simulink model "X31dynamics_03_controller_NDI_MG"  (R2014b)
settings: Solver=ode45  StartTime=0.0  StopTime=30  FixedStep=0.01  RelTol=1e-3
InitFcn:
  | X31dynamics_03_controller_NDI_init
values from neighbouring files (symbols this model uses):
  X31_controller = evalin('base','X31_controller')    [X31dynamics_03_controller_MG_iter_3_2_9_10.m]
undefined symbols (not defined in the file or in its folder): sigbuilder_block, X31_initC, X31_MnvrGen
libraries: simulink x17, QuaternionLib x3
(part 2 of 2)

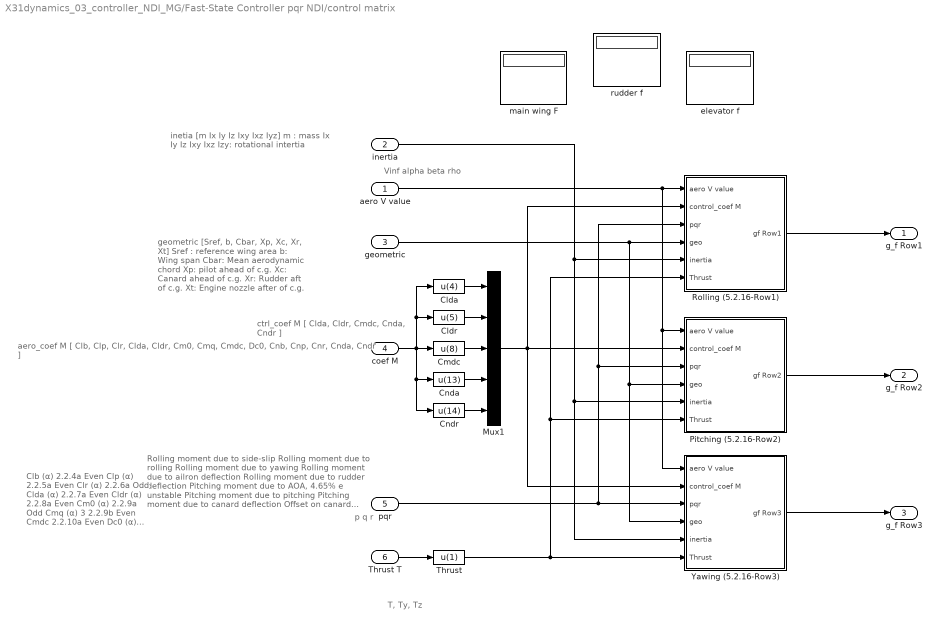
== system X31dynamics_03_controller_NDI_MG/Fast-State Controller pqr NDI/control matrix ==
  note: Vinf alpha beta rho
  note: p q r
  note: geometric
      |  [Sref, b, Cbar, Xp, Xc, Xr, Xt]
      |
      | Sref : reference wing area
      | b: Wing span
      | Cbar: Mean aerodynamic chord
      | Xp: pilot ahead of c.g.
      | Xc: Canard ahead of c.g.
      | Xr: Rudder aft of c.g.
      | Xt: Engine nozzle after of c.g.
  note: Rolling moment due to side-slip
      | Rolling moment due to rolling
      | Rolling moment due to yawing
      | Rolling moment due to ailron deflection
      | Rolling moment due to rudder deflection
      |
      | Pitching moment due to AOA, 4.65% e unstable
      | Pitching moment due to pitching
      | Pitching moment due to canard deflection
      | Offset on canard deflection
      |
      | Yawing moment due to side-slip
      | Yawing moment due to rolling
      | Yawing moment due to yawing
      | Yawing moment due to ailron deflection
      | Yawing moment due to rudder deflection
  note: Clb    (α) 2.2.4a Even
      | Clp    (α) 2.2.5a Even
      | Clr     (α) 2.2.6a Odd
      | Clda  (α) 2.2.7a Even
      | Cldr   (α) 2.2.8a Even
      |
      | Cm0  (α) 2.2.9a Odd
      | Cmq  (α) 3 2.2.9b Even
      | Cmdc      2.2.10a Even
      | Dc0   (α) 2.2.2/10b Odd
      |
      | Cnb  (α) 2.2.4b Even
      | Cnp  (α) 2.2.5b Odd
      | Cnr   (α) 2.2.6b Even
      | Cnda(α) 2.2.7b Even
      | Cndr (α) 2.2.8b Even
  note: aero_coef M
      | [ Clb, Clp, Clr, Clda, Cldr, Cm0, Cmq, Cmdc, Dc0, Cnb, Cnp, Cnr, Cnda, Cndr ]
  note: inetia
      | [m Ix Iy Iz Ixy Ixz Iyz]
      | m : mass
      | Ix Iy Iz Ixy Ixz Izy: rotational intertia
  note: ctrl_coef M
      | [ Clda, Cldr, Cmdc, Cnda, Cndr ]
  note: T, Ty, Tz
  aero V value : Inport
  inertia : Inport  Port=2
  geometric : Inport  Port=3
  coef M : Inport  Port=4
  pqr : Inport  Port=5
  Thrust T : Inport  Port=6
  Clda : Fcn  Expr=u(4)
  Cldr : Fcn  Expr=u(5)
  Cmdc : Fcn  Expr=u(8)
  Cnda : Fcn  Expr=u(13)
  Cndr : Fcn  Expr=u(14)
  Mux1 : Mux  Inputs=5
  Pitching (5.2.16-Row2) : Subsystem
  Rolling (5.2.16-Row1) : Subsystem
  Thrust : Fcn  Expr=u(1)
  Yawing (5.2.16-Row3) : Subsystem
  elevator f : Display
  main wing F : Display
  rudder f : Display
  g_f Row1 : Outport
  g_f Row2 : Outport  Port=2
  g_f Row3 : Outport  Port=3
  wires:
  pqr/1 -> Yawing (5.2.16-Row3)/3(pqr), Pitching (5.2.16-Row2)/3(pqr), Rolling (5.2.16-Row1)/3(pqr)
  aero V value/1 -> Yawing (5.2.16-Row3)/1(aero V value), Pitching (5.2.16-Row2)/1(aero V value), Rolling (5.2.16-Row1)/1(aero V value)
  coef M/1 -> Clda/1, Cldr/1, Cndr/1, Cnda/1, Cmdc/1
  Mux1/1 -> Yawing (5.2.16-Row3)/2(control_coef M), Pitching (5.2.16-Row2)/2(control_coef M), Rolling (5.2.16-Row1)/2(control_coef M)
  geometric/1 -> Yawing (5.2.16-Row3)/4(geo), Pitching (5.2.16-Row2)/4(geo), Rolling (5.2.16-Row1)/4(geo)
  Clda/1 -> Mux1/1
  Cldr/1 -> Mux1/2
  Cmdc/1 -> Mux1/3
  Cnda/1 -> Mux1/4
  Cndr/1 -> Mux1/5
  Thrust T/1 -> Thrust/1
  inertia/1 -> Pitching (5.2.16-Row2)/5(inertia), Yawing (5.2.16-Row3)/5(inertia), Rolling (5.2.16-Row1)/5(inertia)
  Yawing (5.2.16-Row3)/1(gf Row3) -> g_f Row3/1
  Pitching (5.2.16-Row2)/1(gf Row2) -> g_f Row2/1
  Rolling (5.2.16-Row1)/1(gf Row1) -> g_f Row1/1
  Thrust/1 -> Yawing (5.2.16-Row3)/6(Thrust), Pitching (5.2.16-Row2)/6(Thrust), Rolling (5.2.16-Row1)/6(Thrust)

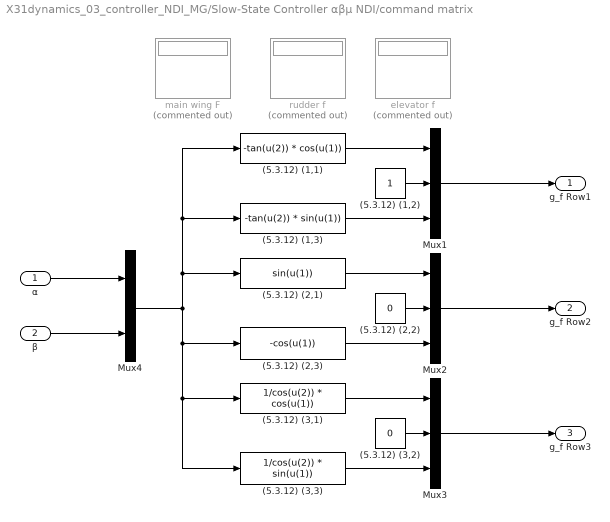
== system X31dynamics_03_controller_NDI_MG/Slow-State Controller αβμ NDI/command matrix ==
  α : Inport
  β : Inport  Port=2
  (5.3.12) (1,1) : Fcn  Expr=-tan(u(2)) * cos(u(1))
  (5.3.12) (1,2) : Constant
  (5.3.12) (1,3) : Fcn  Expr=-tan(u(2)) * sin(u(1))
  (5.3.12) (2,1) : Fcn  Expr=sin(u(1))
  (5.3.12) (2,2) : Constant  Value=0
  (5.3.12) (2,3) : Fcn  Expr=-cos(u(1))
  (5.3.12) (3,1) : Fcn  Expr=1/cos(u(2)) * cos(u(1))
  (5.3.12) (3,2) : Constant  Value=0
  (5.3.12) (3,3) : Fcn  Expr=1/cos(u(2)) * sin(u(1))
  Mux1 : Mux  Inputs=3
  Mux2 : Mux  Inputs=3
  Mux3 : Mux  Inputs=3
  Mux4 : Mux  Inputs=2
  elevator f : Display  Commented=on
  main wing F : Display  Commented=on
  rudder f : Display  Commented=on
  g_f Row1 : Outport
  g_f Row2 : Outport  Port=2
  g_f Row3 : Outport  Port=3
  wires:
  Mux3/1 -> g_f Row3/1
  Mux2/1 -> g_f Row2/1
  Mux1/1 -> g_f Row1/1
  α/1 -> Mux4/1
  β/1 -> Mux4/2
  (5.3.12) (3,2)/1 -> Mux3/2
  (5.3.12) (2,2)/1 -> Mux2/2
  (5.3.12) (1,2)/1 -> Mux1/2
  Mux4/1 -> (5.3.12) (1,3)/1, (5.3.12) (1,1)/1, (5.3.12) (2,1)/1, (5.3.12) (3,3)/1, (5.3.12) (3,1)/1, (5.3.12) (2,3)/1
  (5.3.12) (1,1)/1 -> Mux1/1
  (5.3.12) (1,3)/1 -> Mux1/3
  (5.3.12) (2,1)/1 -> Mux2/1
  (5.3.12) (2,3)/1 -> Mux2/3
  (5.3.12) (3,1)/1 -> Mux3/1
  (5.3.12) (3,3)/1 -> Mux3/3

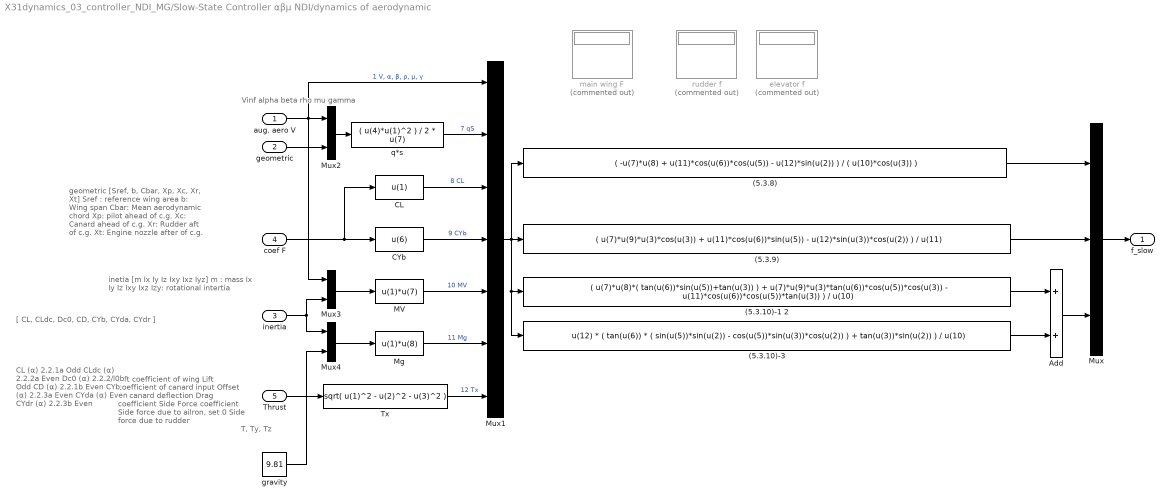
== system X31dynamics_03_controller_NDI_MG/Slow-State Controller αβμ NDI/dynamics of aerodynamic ==
  note: Vinf alpha beta rho mu gamma
  note: geometric
      |  [Sref, b, Cbar, Xp, Xc, Xr, Xt]
      |
      | Sref : reference wing area
      | b: Wing span
      | Cbar: Mean aerodynamic chord
      | Xp: pilot ahead of c.g.
      | Xc: Canard ahead of c.g.
      | Xr: Rudder aft of c.g.
      | Xt: Engine nozzle after of c.g.
  note: Lift coefficient of wing
      | Lift coefficient of canard input
      | Offset on canard deflection
      | Drag coefficient
      | Side Force coefficient
      | Side force due to ailron, set 0
      | Side force due to rudder
  note: CL     (α) 2.2.1a Odd
      | CLdc (α)  2.2.2a Even
      | Dc0   (α)  2.2.2/l0b Odd
      | CD     (α)  2.2.1b Even
      | CYb   (α) 2.2.3a Even
      | CYda (α)            Even
      | CYdr  (α) 2.2.3b Even
  note: [ CL, CLdc, Dc0, CD, CYb, CYda, CYdr ]
  note: T, Ty, Tz
  note: inetia
      | [m Ix Iy Iz Ixy Ixz Iyz]
      | m : mass
      | Ix Iy Iz Ixy Ixz Izy: rotational intertia
  aug. aero V : Inport
  geometric : Inport  Port=2
  inertia : Inport  Port=3
  coef F : Inport  Port=4
  Thrust : Inport  Port=5
  (5.3.10)-1 2 : Fcn  Expr="( u(7)*u(8)*( tan(u(6))*sin(u(5))+tan(u(3)) ) + u(7)*u(9)*u(3)*tan(u(6))*cos(u(5))*cos(u(3)) - u(11)*cos(u(6))*cos(u(5))*tan(u(3)) ) /  u(10)"
  (5.3.10)-3 : Fcn  Expr=u(12) * ( tan(u(6)) * ( sin(u(5))*sin(u(2)) - cos(u(5))*sin(u(3))*cos(u(2)) ) + tan(u(3))*sin(u(2)) ) / u(10)
  (5.3.8) : Fcn  Expr=( -u(7)*u(8) + u(11)*cos(u(6))*cos(u(5)) - u(12)*sin(u(2)) ) / ( u(10)*cos(u(3)) )
  (5.3.9) : Fcn  Expr=( u(7)*u(9)*u(3)*cos(u(3)) + u(11)*cos(u(6))*sin(u(5)) - u(12)*sin(u(3))*cos(u(2)) ) / u(11)
  Add : Sum
  CL : Fcn  Expr=u(1)
  CYb : Fcn  Expr=u(6)
  MV : Fcn  Expr=u(1)*u(7)
  Mg : Fcn  Expr=u(1)*u(8)
  Mux : Mux  Inputs=3
  Mux1 : Mux  Inputs=7
  Mux2 : Mux  Inputs=2
  Mux3 : Mux  Inputs=2
  Mux4 : Mux  Inputs=2
  Tx : Fcn  Expr=sqrt( u(1)^2 - u(2)^2 - u(3)^2 )
  elevator f : Display  Commented=on
  gravity : Constant  Value=9.81
  main wing F : Display  Commented=on
  q*s : Fcn  Expr=( u(4)*u(1)^2 ) / 2 * u(7)
  rudder f : Display  Commented=on
  f_slow : Outport
  wires:
  Mux/1 -> f_slow/1
  aug. aero V/1 -> Mux2/1, Mux1/1, Mux3/1  "1 V, α, β, ρ, μ, γ"
  coef F/1 -> CL/1, CYb/1
  geometric/1 -> Mux2/2
  q*s/1 -> Mux1/2  "7 qS"
  (5.3.10)-1 2/1 -> Add/1
  (5.3.8)/1 -> Mux/1
  (5.3.9)/1 -> Mux/2
  Mux3/1 -> MV/1
  Thrust/1 -> Tx/1
  Tx/1 -> Mux1/7  "12 Tx"
  MV/1 -> Mux1/5  "10 MV"
  CYb/1 -> Mux1/4  "9 CYb"
  CL/1 -> Mux1/3  "8 CL"
  Mux1/1 -> (5.3.8)/1, (5.3.9)/1, (5.3.10)-3/1, (5.3.10)-1 2/1
  Mux2/1 -> q*s/1
  inertia/1 -> Mux4/1, Mux3/2
  Mg/1 -> Mux1/6  "11 Mg"
  Mux4/1 -> Mg/1
  gravity/1 -> Mux4/2
  (5.3.10)-3/1 -> Add/2
  Add/1 -> Mux/3

== system X31dynamics_03_controller_NDI_MG/Fast-State Controller pqr NDI/aerodynamic Moment/Pitching coefficient (5.2.14) ==
  note: 9 p q r
  note: 1 Vinf alpha beta rho
  note: 12 Sref, b, Cbar, Xp, Xc, Xr, Xt
  note: 5 Cm0, Cmq, Cmdc, Dc0
  aero V value : Inport
  aero_coef Mb : Inport  Port=2
  pqr : Inport  Port=3
  geo : Inport  Port=4
  Add : Sum
  Aero : Display
  Mux : Mux
  ail prop F body : Display
  main wing F : Display
  pitching (5.2.14-2) : Fcn  Expr=u(6)* u(10)*u(14) / (2*u(1))
  stateR 2 : Display
  static stability (5.2.14-1) : Fcn  Expr=u(5)
  Cm : Outport
  wires:
  aero_coef Mb/1 -> Mux/2
  Mux/1 -> static stability (5.2.14-1)/1, pitching (5.2.14-2)/1
  aero V value/1 -> Mux/1
  pqr/1 -> Mux/3
  pitching (5.2.14-2)/1 -> Add/2
  static stability (5.2.14-1)/1 -> Add/1
  Add/1 -> Cm/1
  geo/1 -> Mux/4

== system X31dynamics_03_controller_NDI_MG/Fast-State Controller pqr NDI/aerodynamic Moment/Rolling coefficient (5.2.13) ==
  note: 10 p q r
  note: 1 Vinf alpha beta rho
  note: 5 Clb, Clp, Clr, Clda, Cldr
  note: 13 Sref, b, Cbar, Xp, Xc, Xr, Xt
  aero V value : Inport
  aero_coef M : Inport  Port=2
  pqr : Inport  Port=3
  geo : Inport  Port=4
  Add : Sum  Inputs=+++
  Aero : Display  Commented=on
  Mux : Mux
  ail prop F body : Display  Commented=on
  main wing F : Display  Commented=on
  rolling (5.2.13-2) : Fcn  Expr=u(6)* u(10)*u(14) / (2*u(1))
  sideslip (5.2.13-1) : Fcn  Expr=u(5)*u(3)
  stateR 2 : Display  Commented=on
  yawing (5.2.13-3) : Fcn  Expr=u(7)* u(12)*u(14) / (2*u(1))
  Cl hat : Outport
  wires:
  aero_coef M/1 -> Mux/2
  Mux/1 -> sideslip (5.2.13-1)/1, rolling (5.2.13-2)/1, yawing (5.2.13-3)/1
  aero V value/1 -> Mux/1
  pqr/1 -> Mux/3
  geo/1 -> Mux/4
  yawing (5.2.13-3)/1 -> Add/3
  rolling (5.2.13-2)/1 -> Add/2
  sideslip (5.2.13-1)/1 -> Add/1
  Add/1 -> Cl hat/1

== system X31dynamics_03_controller_NDI_MG/Fast-State Controller pqr NDI/aerodynamic Moment/Yawing coefficient (5.2.15) ==
  note: 10 p q r
  note: 1 Vinf alpha beta rho
  note: 13 Sref, b, Cbar, Xp, Xc, Xr, Xt
  note: 5 Cnb, Cnp, Cnr, Cnda, Cndr
  aero V value : Inport
  aero_coef M : Inport  Port=2
  pqr : Inport  Port=3
  geo : Inport  Port=4
  Add : Sum  Inputs=+++
  Aero : Display
  Mux : Mux
  ail prop F body : Display
  main wing F : Display
  rolling (5.2.15-2) : Fcn  Expr=u(6)* u(10)*u(14) / (2*u(1))
  sideslip (5.2.15-1) : Fcn  Expr=u(5)*u(3)
  stateR 2 : Display
  yawing (5.2.15-3) : Fcn  Expr=u(7)* u(10)*u(12) / (2*u(1))
  Cn : Outport
  wires:
  aero_coef M/1 -> Mux/2
  Mux/1 -> ail prop F body/1, sideslip (5.2.15-1)/1, rolling (5.2.15-2)/1, yawing (5.2.15-3)/1
  aero V value/1 -> stateR 2/1, Mux/1
  pqr/1 -> Mux/3
  geo/1 -> Mux/4
  yawing (5.2.15-3)/1 -> Add/3
  rolling (5.2.15-2)/1 -> main wing F/1, Add/2
  sideslip (5.2.15-1)/1 -> Add/1
  Add/1 -> Cn/1

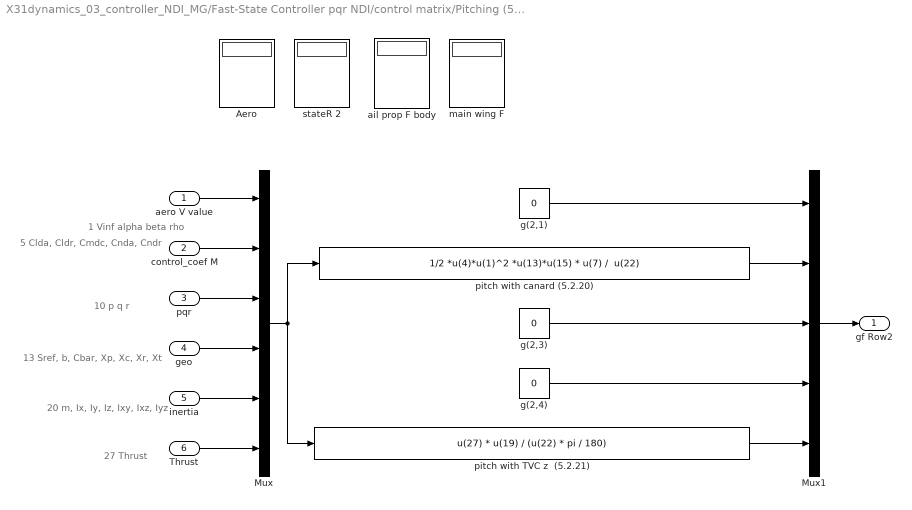
== system X31dynamics_03_controller_NDI_MG/Fast-State Controller pqr NDI/control matrix/Pitching (5.2.16-Row2) ==
  note: 27 Thrust
  note: 10 p q r
  note: 1 Vinf alpha beta rho
  note: 13 Sref, b, Cbar, Xp, Xc, Xr, Xt
  note: 20 m, Ix, Iy, Iz, Ixy, Ixz, Iyz
  note: 5 Clda, Cldr, Cmdc, Cnda, Cndr
  aero V value : Inport
  control_coef M : Inport  Port=2
  pqr : Inport  Port=3
  geo : Inport  Port=4
  inertia : Inport  Port=5
  Thrust : Inport  Port=6
  Aero : Display
  Mux : Mux  Inputs=6
  Mux1 : Mux  Inputs=5
  ail prop F body : Display
  g(2,1) : Constant  Value=0
  g(2,3) : Constant  Value=0
  g(2,4) : Constant  Value=0
  main wing F : Display
  pitch with TVC z  (5.2.21) : Fcn  Expr=u(27) * u(19) / (u(22) * pi / 180)
  pitch with canard (5.2.20) : Fcn  Expr="1/2 *u(4)*u(1)^2 *u(13)*u(15) * u(7) /  u(22)"
  stateR 2 : Display
  gf Row2 : Outport
  wires:
  control_coef M/1 -> Mux/2
  Mux/1 -> pitch with TVC z  (5.2.21)/1, pitch with canard (5.2.20)/1
  aero V value/1 -> Mux/1
  pqr/1 -> Mux/3
  geo/1 -> Mux/4
  pitch with TVC z  (5.2.21)/1 -> Mux1/5
  g(2,3)/1 -> Mux1/3
  pitch with canard (5.2.20)/1 -> Mux1/2
  Mux1/1 -> gf Row2/1
  g(2,1)/1 -> Mux1/1
  g(2,4)/1 -> Mux1/4
  inertia/1 -> Mux/5
  Thrust/1 -> Mux/6

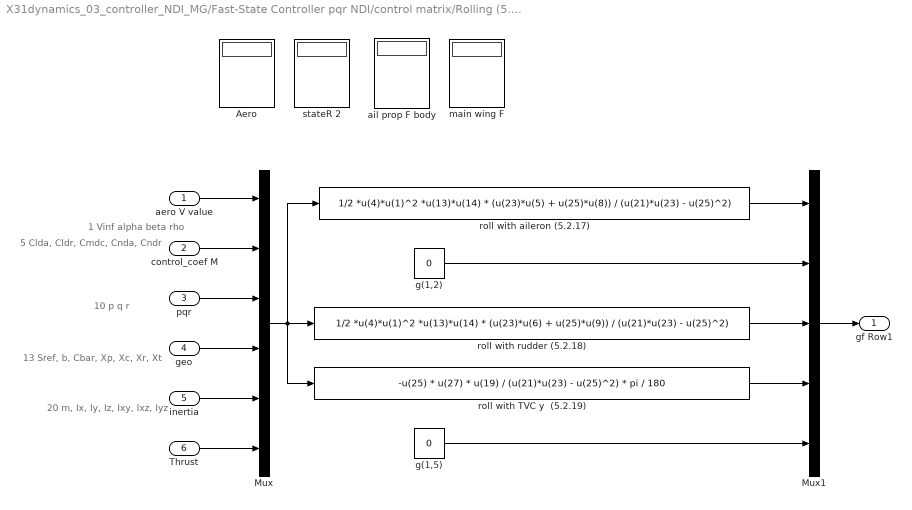
== system X31dynamics_03_controller_NDI_MG/Fast-State Controller pqr NDI/control matrix/Rolling (5.2.16-Row1) ==
  note: 10 p q r
  note: 1 Vinf alpha beta rho
  note: 13 Sref, b, Cbar, Xp, Xc, Xr, Xt
  note: 20 m, Ix, Iy, Iz, Ixy, Ixz, Iyz
  note: 5 Clda, Cldr, Cmdc, Cnda, Cndr
  aero V value : Inport
  control_coef M : Inport  Port=2
  pqr : Inport  Port=3
  geo : Inport  Port=4
  inertia : Inport  Port=5
  Thrust : Inport  Port=6
  Aero : Display
  Mux : Mux  Inputs=6
  Mux1 : Mux  Inputs=5
  ail prop F body : Display
  g(1,2) : Constant  Value=0
  g(1,5) : Constant  Value=0
  main wing F : Display
  roll with TVC y  (5.2.19) : Fcn  Expr=-u(25) * u(27) * u(19) / (u(21)*u(23) - u(25)^2) * pi / 180
  roll with aileron (5.2.17) : Fcn  Expr=1/2 *u(4)*u(1)^2 *u(13)*u(14) * (u(23)*u(5) + u(25)*u(8)) / (u(21)*u(23) - u(25)^2)
  roll with rudder (5.2.18) : Fcn  Expr=1/2 *u(4)*u(1)^2 *u(13)*u(14) * (u(23)*u(6) + u(25)*u(9)) / (u(21)*u(23) - u(25)^2)
  stateR 2 : Display
  gf Row1 : Outport
  wires:
  control_coef M/1 -> Mux/2
  Mux/1 -> roll with rudder (5.2.18)/1, roll with TVC y  (5.2.19)/1, roll with aileron (5.2.17)/1
  aero V value/1 -> Mux/1
  pqr/1 -> Mux/3
  geo/1 -> Mux/4
  roll with TVC y  (5.2.19)/1 -> Mux1/4
  roll with rudder (5.2.18)/1 -> Mux1/3
  roll with aileron (5.2.17)/1 -> Mux1/1
  Mux1/1 -> gf Row1/1
  g(1,2)/1 -> Mux1/2
  g(1,5)/1 -> Mux1/5
  inertia/1 -> Mux/5
  Thrust/1 -> Mux/6

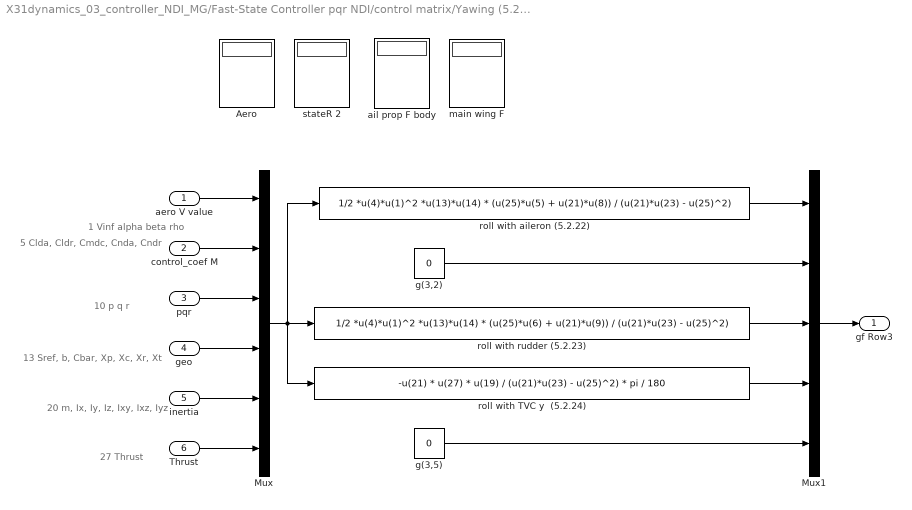
== system X31dynamics_03_controller_NDI_MG/Fast-State Controller pqr NDI/control matrix/Yawing (5.2.16-Row3) ==
  note: 27 Thrust
  note: 10 p q r
  note: 1 Vinf alpha beta rho
  note: 13 Sref, b, Cbar, Xp, Xc, Xr, Xt
  note: 20 m, Ix, Iy, Iz, Ixy, Ixz, Iyz
  note: 5 Clda, Cldr, Cmdc, Cnda, Cndr
  aero V value : Inport
  control_coef M : Inport  Port=2
  pqr : Inport  Port=3
  geo : Inport  Port=4
  inertia : Inport  Port=5
  Thrust : Inport  Port=6
  Aero : Display
  Mux : Mux  Inputs=6
  Mux1 : Mux  Inputs=5
  ail prop F body : Display
  g(3,2) : Constant  Value=0
  g(3,5) : Constant  Value=0
  main wing F : Display
  roll with TVC y  (5.2.24) : Fcn  Expr=-u(21) * u(27) * u(19) / (u(21)*u(23) - u(25)^2) * pi / 180
  roll with aileron (5.2.22) : Fcn  Expr=1/2 *u(4)*u(1)^2 *u(13)*u(14) * (u(25)*u(5) + u(21)*u(8)) / (u(21)*u(23) - u(25)^2)
  roll with rudder (5.2.23) : Fcn  Expr=1/2 *u(4)*u(1)^2 *u(13)*u(14) * (u(25)*u(6) + u(21)*u(9)) / (u(21)*u(23) - u(25)^2)
  stateR 2 : Display
  gf Row3 : Outport
  wires:
  control_coef M/1 -> Mux/2
  Mux/1 -> roll with rudder (5.2.23)/1, roll with TVC y  (5.2.24)/1, roll with aileron (5.2.22)/1
  aero V value/1 -> Mux/1
  pqr/1 -> Mux/3
  geo/1 -> Mux/4
  roll with TVC y  (5.2.24)/1 -> Mux1/4
  roll with rudder (5.2.23)/1 -> Mux1/3
  roll with aileron (5.2.22)/1 -> Mux1/1
  Mux1/1 -> gf Row3/1
  g(3,2)/1 -> Mux1/2
  g(3,5)/1 -> Mux1/5
  inertia/1 -> Mux/5
  Thrust/1 -> Mux/6

== matlab function X31dynamics_03_controller_NDI_MG/coefficient/aerodynamic coefficient ==
  data: fa output; a input; fb output; X31_controller parameter
function [fa,fb] = aero_coef(a,X31_controller) 
X31_controller_aero_poly = X31_controller.aero_poly;
    fa = zeros(1,10);
    fb = zeros(1,10);
    a = 180 / pi * a;   % convert to degree for polynomials
    a_abs = abs(a);
    for i = 1:10
        fa(i) = X31_controller_aero_poly.fig2_2(i).a(6)*a_abs^6 + X31_controller_aero_poly.fig2_2(i).a(5)*a_abs^5 + X31_controller_aero_poly.fig2_2(i).a(4)*a_abs^4 +...
                X31_controller_aero_poly.fig2_2(i).a(3)*a_abs^3 + X31_controller_aero_poly.fig2_2(i).a(2)*a_abs^2 + X31_controller_aero_poly.fig2_2(i).a(1)*a_abs + X31_controller_aero_poly.fig2_2(i).a(7);

        fb(i) = X31_controller_aero_poly.fig2_2(i).b(6)*a_abs^6 + X31_controller_aero_poly.fig2_2(i).b(5)*a_abs^5 + X31_controller_aero_poly.fig2_2(i).b(4)*a_abs^4 +...
                X31_controller_aero_poly.fig2_2(i).b(3)*a_abs^3 + X31_controller_aero_poly.fig2_2(i).b(2)*a_abs^2 + X31_controller_aero_poly.fig2_2(i).b(1)*a_abs + X31_controller_aero_poly.fig2_2(i).b(7);
        % for odd functions
        if (a<0) 
            if (X31_controller_aero_poly.fig2_2(i).a(8) ==1)
                fa(i) = -fa(i) + 2*X31_controller_aero_poly.fig2_2(i).a(7);
            end
            if (X31_controller_aero_poly.fig2_2(i).b(8) ==1)
                fb(i) = -fb(i) + 2*X31_controller_aero_poly.fig2_2(i).b(7);
            end
        end
    end
end

%{
     Force
CL   (α) 2.2.1a Odd
CLdc (α) 2.2.2a Even
C0d  (α) 2.2.2/l0b Odd
CD   (α) 2.2.1b Even
CYp  (α) 2.2.3a Even
CYda (α) Set zero Not Shown Even
CYdr (α) 2.2.3b Even

     Moment
Clb  (α) 2.2.4a Even
Clp  (α) 2.2.5a Even
Clr  (α) 2.2.6a Odd
Clda (α) 2.2.7a Even
Cldr (α) 2.2.8a Even

Cm0  (α) 4.65% e unstable 2.2.9a Odd
Cmq  (α) 3 2.2.9b Even
Cmdc      2.2.10a Even
C0d  (α) 2.2.2/10b Odd

Cnb  (α) 2.2.4b Even
Cnp  (α) 2.2.5b Odd
Cnr  (α) 2.2.6b Even
Cnda (α) 2.2.7b Even
Cndr (α) 2.2.8b Even
%}

== matlab function X31dynamics_03_controller_NDI_MG/Fast-State Controller pqr NDI/(5.2.9) f_fast ==
  data: inertia input; f output size=3; moments input; pqr input
function f = NDI_f_fast(inertia, moments, pqr)
Ixx = inertia(2);
Iyy = inertia(3);
Izz = inertia(4);
Ixz = inertia(6);
p = pqr(1);
q = pqr(2);
r = pqr(3);
l = moments(1);
m = moments(2);
n = moments(3);

f = zeros(3,1);
f(1) = (Izz*l + Ixz*n) / (Ixx*Izz - Ixz^2) + ( Ixz*(Ixx - Iyy + Izz)*p*q + (Izz*(Iyy - Izz) - Ixz^2)*q*r ) / (Ixx*Izz - Ixz^2);
f(2) = m / Iyy + ((Izz - Ixx)*p*r + Ixz*(r^2-p^2)) / Iyy;
f(3) = (Ixz*l + Ixx*n) / (Ixx*Izz - Ixz^2) + ( (Ixx*(Ixx - Iyy) - Ixz^2)*p*q - Ixz*(Ixx - Iyy + Izz)*q*r ) / (Ixx*Izz - Ixz^2);
end

== matlab function X31dynamics_03_controller_NDI_MG/Fast-State Controller pqr NDI/(5.2.36) ==
  data: y_bar input; aileron output; g_row1 input; g_row2 input; g_row3 input; canard output; rudder output; TVC_y output; TVC_z output
function [aileron, canard, rudder, TVC_y, TVC_z] = NDI(y_bar, g_row1, g_row2, g_row3)
g_f = zeros(3,5);
g_f(1,1:5) = g_row1;
g_f(2,1:5) = g_row2;
g_f(3,1:5) = g_row3;

delta_max = diag([30, 30, 30, 15, 15]);         % by (5.2.41)
gt_f = g_f * delta_max;                       % by (5.2.43)
pseudo_inv_gt_f = gt_f'/(gt_f*gt_f');           % by (5.2.37)
u_bar = (delta_max*pseudo_inv_gt_f)*y_bar;      % (5.2.45) to (5.2.36)

aileron = u_bar(1);
canard = u_bar(2);
rudder = u_bar(3);
TVC_y = u_bar(4);
TVC_z = u_bar(5);
end

== matlab function X31dynamics_03_controller_NDI_MG/Slow-State Controller αβμ NDI/(5.3.29) ==
  data: y_bar input; p_c output; g_row1 input; g_row2 input; g_row3 input; q_c output; r_c output
function [p_c, q_c, r_c] = NDI(y_bar, g_row1, g_row2, g_row3)
g_s = zeros(3,3);
g_s(1,1:3) = g_row1;
g_s(2,1:3) = g_row2;
g_s(3,1:3) = g_row3;


u_bar = g_s \ y_bar;      % (5.2.45) to (5.2.36)
p_c = u_bar(1);
q_c = u_bar(2);
r_c = u_bar(3);
end
